simulink subsystem "trajectory_generation_ref_subsys_7dof"  (R2022b)
settings: Solver=VariableStepAuto  StartTime=0.0  StopTime=10.0  RelTol=1e-3
undefined symbols (not defined in the file): init_bus_param, param_traj
settings Model: Creator=emu  LastModifiedBy=emu
settings OptimizationCC: ReuseModelBlockBuffer=on

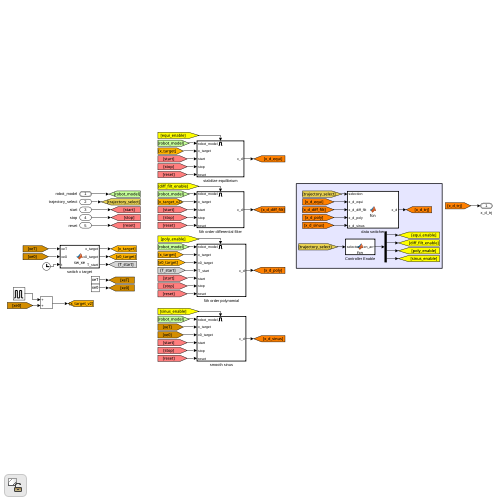
[thumbnail: Simulink's stored preview of the top-level diagram]
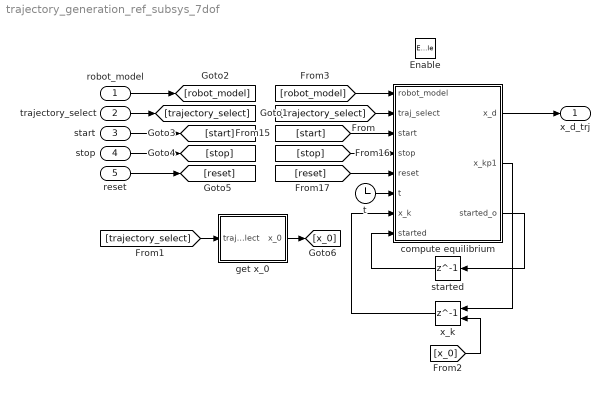
== system trajectory_generation_ref_subsys_7dof ==
  robot_model : Inport  OutDataTypeStr=Bus: robot_model
  trajectory_select : Inport  Port=2
  start : Inport  Port=3
  stop : Inport  Port=4
  reset : Inport  Port=5
  Enable : EnablePort
  compute equilibrium : MATLAB Function  TreatAsAtomicUnit=on
  get x_0 : MATLAB Function  TreatAsAtomicUnit=on
  started : Delay  DelayLength=1
  t : Clock
  x_k : Delay  DelayLength=1  InitialConditionSource=Input port  InitialCondition=[param_traj.pose.xe0(1);0;0;0;0;0; param_traj.pose.xe0(2);0;0;0;0;0; param_traj.pose.xe0(3);0;0;0;0;0; param_traj.pose.alpha0;0;0;0;0;0];
      settings: InputPortMap=u0,p4
  x_d_trj : Outport  OutDataTypeStr=Bus: x_d
  wires:
  stop/1 -> [stop]
  start/1 -> [start]
  reset/1 -> [reset]
  compute equilibrium/1(x_d) -> x_d_trj/1
  robot_model/1 -> [robot_model]
  trajectory_select/1 -> [trajectory_select]
  x_k/1 -> compute equilibrium/7(x_k)
  [start] -> compute equilibrium/3(start)
  [trajectory_select] -> compute equilibrium/2(traj_select)
  compute equilibrium/2(x_kp1) -> x_k/1
  [reset] -> compute equilibrium/5(reset)
  started/1 -> compute equilibrium/8(started)
  compute equilibrium/3(started_o) -> started/1
  [robot_model] -> compute equilibrium/1(robot_model)
  [stop] -> compute equilibrium/4(stop)
  t/1 -> compute equilibrium/6(t)
  [trajectory_select] -> get x_0/1(traj_select)
  get x_0/1(x_0) -> [x_0]
  [x_0] -> x_k/2

== matlab function trajectory_generation_ref_subsys_7dof/get x_0 ==
  data: traj_select input; x_0 output; param_traj parameter
function x_0 = fcn(traj_select, param_traj)
    start_index = param_traj.traj_init.start_index(traj_select);
    xe0 = param_traj.traj_init.pose(1:3, start_index);
    alpha0 = param_traj.traj_init.alpha(start_index);

    x_0 = [ xe0(1); 0; 0; 0; 0; 0; ...
            xe0(2); 0; 0; 0; 0; 0; ...
            xe0(3); 0; 0; 0; 0; 0; ...
            alpha0; 0; 0; 0; 0; 0 ];

== matlab function trajectory_generation_ref_subsys_7dof/compute equilibrium ==
  settings: updateMethod=DISCRETE  sampleTime=param_global.Ta
  data: robot_model input Bus: robot_model; traj_select input; start input; stop input; reset input; t input; x_k input; x_d output Bus: x_d; x_kp1 output; started input; param_traj parameter; started_o output; init_bus_param parameter


function [x_d, x_kp1, started_o] = ss_z(robot_model, traj_select, start, stop, reset, t, x_k, started, param_traj, init_bus_param)

if(reset == 1 || stop == 1)
    started = 0;
    start_index = param_traj.traj_init.start_index(traj_select);
    xe0 = param_traj.traj_init.pose(1:3, start_index);
    alpha0 = param_traj.traj_init.alpha(start_index);

    x_k = [ xe0(1); 0; 0; 0; 0; 0; ...
            xe0(2); 0; 0; 0; 0; 0; ...
            xe0(3); 0; 0; 0; 0; 0; ...
            alpha0; 0; 0; 0; 0; 0 ];
end

if(start == 1 && stop == 0 && ~started)
    started = 1;
end

if(started == 1)
    if(traj_select == 1)
        [x_d] = create_equilibrium_traj(traj_select, t, param_traj, init_bus_param);
        x_kp1 = x_k;
    elseif(traj_select == 2)
        [x_d, x_kp1] = create_diff_filter_traj(traj_select, t, x_k, param_traj, init_bus_param);
    elseif(traj_select == 3)
        [x_d] = create_poly_traj(traj_select, t, param_traj, init_bus_param);
        x_kp1 = x_k;
    else % trajectory_select == 4
        [x_d] = create_sinus_traj(traj_select, t, param_traj, init_bus_param);
        x_kp1 = x_k;
    end
else
    x_kp1 = x_k;

    H = robot_model.H;
    p_e = H(1:3, 4);
    R_e = H(1:3, 1:3);

    x_d = init_bus_param.x_d;
    x_d.p_d   = p_e;
    x_d.Phi_d = rotm2eul_v2(R_e);
    x_d.R_d   = R_e;
    x_d.q_d   = rotm2quat_v4(R_e);
end

started_o = started;
